simulink model "trainGate"  (R2014b)
settings: Solver=ode1  StartTime=0.0  StopTime=100  FixedStep=0.0001  MaxStep=0.0001  RelTol=1e-3
(part 1 of 2)
settings Model: Creator=sand080  LastModifiedBy=nall426
settings DataIOCC: LimitDataPoints=off
settings RTWCC: CustomInitializer=gettimeofday(&t0, 0);
settings RTWCC: CustomSourceCode=|
  | int gettimeofday(struct timeval * tp, struct timezone * tzp)
  | {
  |     // Note: some broken versions only have 8 trailing zero's, the correct epoch has 9 trailing zero's
  |     static const uint64_t EPOCH = ((uint64_t) 116444736000000000ULL);
  | 
  |     SYSTEMTIME  system_time;
  |     FILETIME    file_time;
  |     uint64_t    time;
  | 
  | 	GetSystemTime( &system_time );
  |     SystemTimeToFileTime( &system_time, &file_time );
  |     time =  ((uint64_t)file_time.dwLowDateTime )      ;
  |     time += ((uint64_t)file_time.dwHighDateTime) << 32;
  | 
  |     tp->tv_sec  = (long) ((time - EPOCH) / 10000000L);
  |     tp->tv_usec = (long) (system_time.wMilliseconds * 1000);
  |     return 0;
  | }
  | 
  | struct timeval t0, t1;
settings RTWCC: CustomHeaderCode=|
  | #include <stdint.h> // portable: uint64_t   MSVC: __int64
  | #include <Windows.h>
settings RTWCC: CustomTerminator=|
  | gettimeofday(&t1, 0);
  | 
  | long elapsed = (t1.tv_sec-t0.tv_sec)*1000000 + t1.tv_usec-t0.tv_usec;
  | printf("Time taken: %ld microseconds (%.3f seconds)\n", elapsed, (elapsed / 1000000.0));

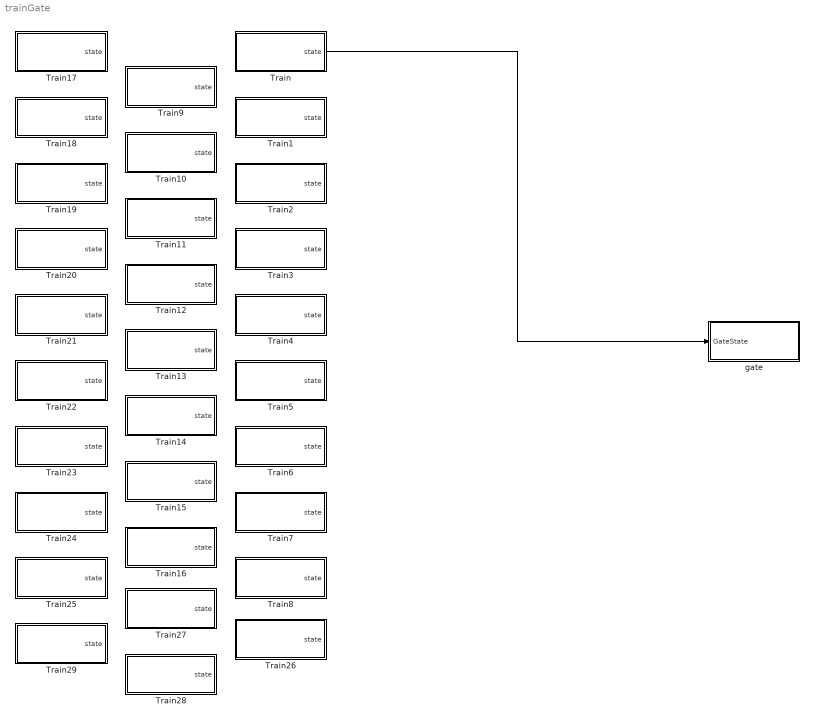
== system trainGate ==
  Train : Subsystem
  Train1 : Subsystem
  Train10 : Subsystem
  Train11 : Subsystem
  Train12 : Subsystem
  Train13 : Subsystem
  Train14 : Subsystem
  Train15 : Subsystem
  Train16 : Subsystem
  Train17 : Subsystem
  Train18 : Subsystem
  Train19 : Subsystem
  Train2 : Subsystem
  Train20 : Subsystem
  Train21 : Subsystem
  Train22 : Subsystem
  Train23 : Subsystem
  Train24 : Subsystem
  Train25 : Subsystem
  Train26 : Subsystem
  Train27 : Subsystem
  Train28 : Subsystem
  Train29 : Subsystem
  Train3 : Subsystem
  Train4 : Subsystem
  Train5 : Subsystem
  Train6 : Subsystem
  Train7 : Subsystem
  Train8 : Subsystem
  Train9 : Subsystem
  gate : Subsystem
  wires:
  Train/1(state) -> gate/1(GateState)

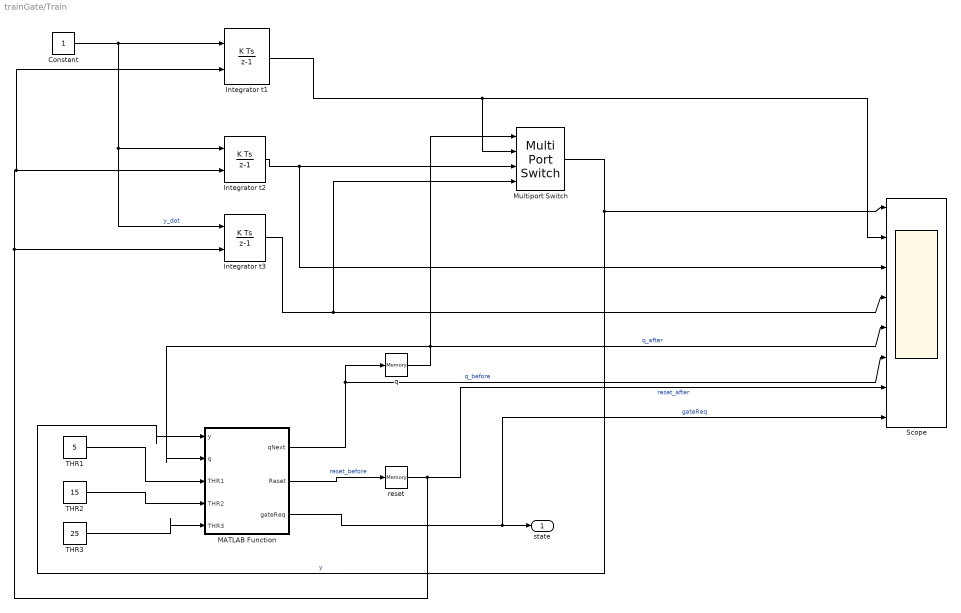
== system trainGate/Train ==
  Constant : Constant
  Integrator t1 : DiscreteIntegrator  ExternalReset=either  InitialConditionSetting=State (most efficient)  SampleTime=-1
  Integrator t2 : DiscreteIntegrator  ExternalReset=either  InitialCondition=5  InitialConditionSetting=State (most efficient)  SampleTime=-1
  Integrator t3 : DiscreteIntegrator  ExternalReset=either  InitialCondition=15  InitialConditionSetting=State (most efficient)  SampleTime=-1
  MATLAB Function : MATLAB Function  Priority=1  TreatAsAtomicUnit=on
  Multiport Switch : MultiPortSwitch
  Scope : Scope  NumInputPorts=8
      settings: TickLabels=on  ShowLegends=on  YMin=0~0~0~10~1~1~0~-1  YMax=40~20~20~30~3~3~1~1
  THR1 : Constant  Value=5
  THR2 : Constant  Value=15
  THR3 : Constant  Value=25
  q : Memory  X0=1  LinearizeMemory=on
  reset : Memory  X0=1  LinearizeMemory=on
  state : Outport
  wires:
  MATLAB Function/1(qNext) -> q/1, Scope/6  "q_before"
  Constant/1 -> Integrator t2/1, Integrator t3/1, Integrator t1/1  "y_dot"
  Integrator t2/1 -> Multiport Switch/3, Scope/3
  Integrator t1/1 -> Scope/2, Multiport Switch/2
  THR1/1 -> MATLAB Function/3(THR1)
  THR2/1 -> MATLAB Function/4(THR2)
  q/1 -> Multiport Switch/1, MATLAB Function/2(q), Scope/5  "q_after"
  THR3/1 -> MATLAB Function/5(THR3)
  Integrator t3/1 -> Multiport Switch/4, Scope/4
  MATLAB Function/2(Reset) -> reset/1  "reset_before"
  Multiport Switch/1 -> Scope/1, MATLAB Function/1(y)  "y"
  reset/1 -> Integrator t1/2, Integrator t2/2, Integrator t3/2, Scope/7  "reset_after"
  MATLAB Function/3(gateReq) -> Scope/8, state/1  "gateReq"

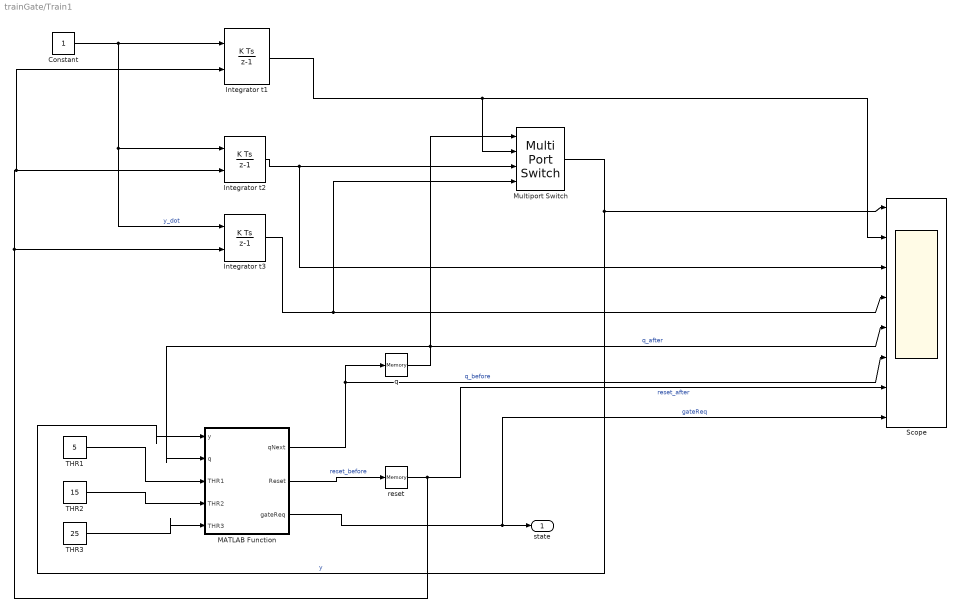
== system trainGate/Train1 ==
  Constant : Constant
  Integrator t1 : DiscreteIntegrator  ExternalReset=either  InitialConditionSetting=State (most efficient)  SampleTime=-1
  Integrator t2 : DiscreteIntegrator  ExternalReset=either  InitialCondition=5  InitialConditionSetting=State (most efficient)  SampleTime=-1
  Integrator t3 : DiscreteIntegrator  ExternalReset=either  InitialCondition=15  InitialConditionSetting=State (most efficient)  SampleTime=-1
  MATLAB Function : MATLAB Function  Priority=1  TreatAsAtomicUnit=on
  Multiport Switch : MultiPortSwitch
  Scope : Scope  NumInputPorts=8
      settings: TickLabels=on  ShowLegends=on  YMin=0~0~0~10~1~1~0~-1  YMax=40~20~20~30~3~3~1~1
  THR1 : Constant  Value=5
  THR2 : Constant  Value=15
  THR3 : Constant  Value=25
  q : Memory  X0=1  LinearizeMemory=on
  reset : Memory  X0=1  LinearizeMemory=on
  state : Outport
  wires:
  MATLAB Function/1(qNext) -> q/1, Scope/6  "q_before"
  Constant/1 -> Integrator t2/1, Integrator t3/1, Integrator t1/1  "y_dot"
  Integrator t2/1 -> Multiport Switch/3, Scope/3
  Integrator t1/1 -> Scope/2, Multiport Switch/2
  THR1/1 -> MATLAB Function/3(THR1)
  THR2/1 -> MATLAB Function/4(THR2)
  q/1 -> Multiport Switch/1, MATLAB Function/2(q), Scope/5  "q_after"
  THR3/1 -> MATLAB Function/5(THR3)
  Integrator t3/1 -> Multiport Switch/4, Scope/4
  MATLAB Function/2(Reset) -> reset/1  "reset_before"
  Multiport Switch/1 -> Scope/1, MATLAB Function/1(y)  "y"
  reset/1 -> Integrator t1/2, Integrator t2/2, Integrator t3/2, Scope/7  "reset_after"
  MATLAB Function/3(gateReq) -> Scope/8, state/1  "gateReq"

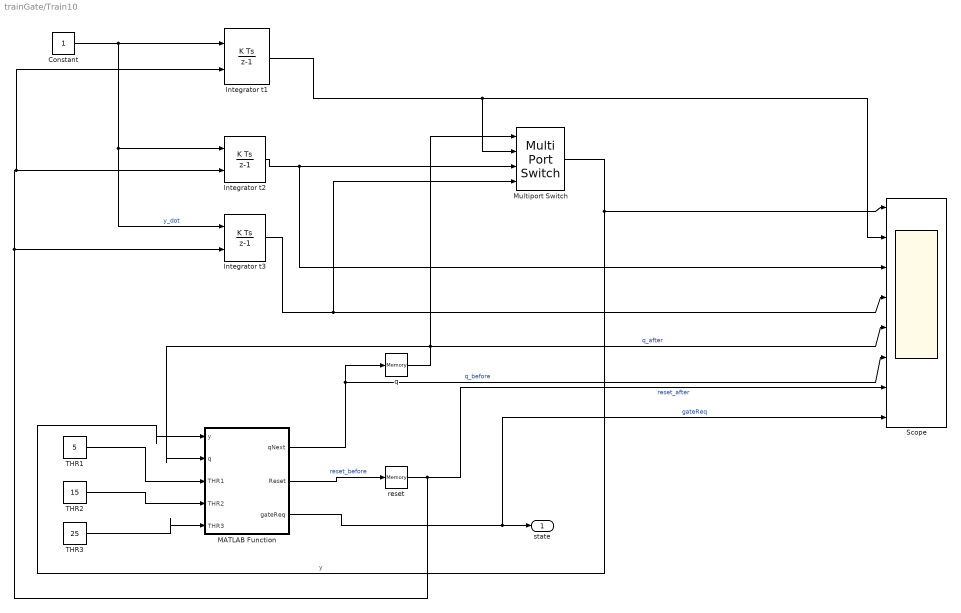
== system trainGate/Train10 ==
  Constant : Constant
  Integrator t1 : DiscreteIntegrator  ExternalReset=either  InitialConditionSetting=State (most efficient)  SampleTime=-1
  Integrator t2 : DiscreteIntegrator  ExternalReset=either  InitialCondition=5  InitialConditionSetting=State (most efficient)  SampleTime=-1
  Integrator t3 : DiscreteIntegrator  ExternalReset=either  InitialCondition=15  InitialConditionSetting=State (most efficient)  SampleTime=-1
  MATLAB Function : MATLAB Function  Priority=1  TreatAsAtomicUnit=on
  Multiport Switch : MultiPortSwitch
  Scope : Scope  NumInputPorts=8
      settings: TickLabels=on  ShowLegends=on  YMin=0~0~0~10~1~1~0~-1  YMax=40~20~20~30~3~3~1~1
  THR1 : Constant  Value=5
  THR2 : Constant  Value=15
  THR3 : Constant  Value=25
  q : Memory  X0=1  LinearizeMemory=on
  reset : Memory  X0=1  LinearizeMemory=on
  state : Outport
  wires:
  MATLAB Function/1(qNext) -> q/1, Scope/6  "q_before"
  Constant/1 -> Integrator t2/1, Integrator t3/1, Integrator t1/1  "y_dot"
  Integrator t2/1 -> Multiport Switch/3, Scope/3
  Integrator t1/1 -> Scope/2, Multiport Switch/2
  THR1/1 -> MATLAB Function/3(THR1)
  THR2/1 -> MATLAB Function/4(THR2)
  q/1 -> Multiport Switch/1, MATLAB Function/2(q), Scope/5  "q_after"
  THR3/1 -> MATLAB Function/5(THR3)
  Integrator t3/1 -> Multiport Switch/4, Scope/4
  MATLAB Function/2(Reset) -> reset/1  "reset_before"
  Multiport Switch/1 -> Scope/1, MATLAB Function/1(y)  "y"
  reset/1 -> Integrator t1/2, Integrator t2/2, Integrator t3/2, Scope/7  "reset_after"
  MATLAB Function/3(gateReq) -> Scope/8, state/1  "gateReq"

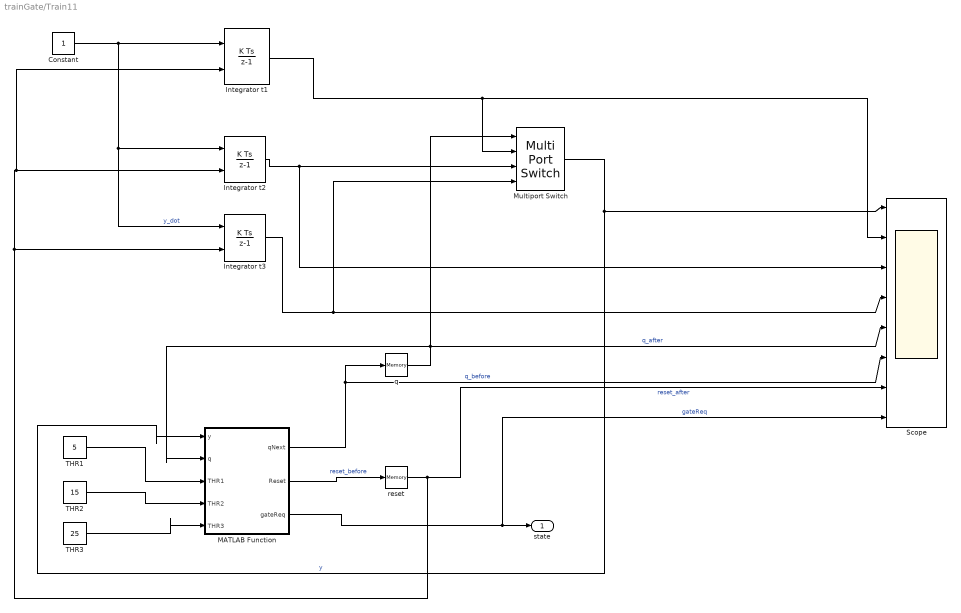
== system trainGate/Train11 ==
  Constant : Constant
  Integrator t1 : DiscreteIntegrator  ExternalReset=either  InitialConditionSetting=State (most efficient)  SampleTime=-1
  Integrator t2 : DiscreteIntegrator  ExternalReset=either  InitialCondition=5  InitialConditionSetting=State (most efficient)  SampleTime=-1
  Integrator t3 : DiscreteIntegrator  ExternalReset=either  InitialCondition=15  InitialConditionSetting=State (most efficient)  SampleTime=-1
  MATLAB Function : MATLAB Function  Priority=1  TreatAsAtomicUnit=on
  Multiport Switch : MultiPortSwitch
  Scope : Scope  NumInputPorts=8
      settings: TickLabels=on  ShowLegends=on  YMin=0~0~0~10~1~1~0~-1  YMax=40~20~20~30~3~3~1~1
  THR1 : Constant  Value=5
  THR2 : Constant  Value=15
  THR3 : Constant  Value=25
  q : Memory  X0=1  LinearizeMemory=on
  reset : Memory  X0=1  LinearizeMemory=on
  state : Outport
  wires:
  MATLAB Function/1(qNext) -> q/1, Scope/6  "q_before"
  Constant/1 -> Integrator t2/1, Integrator t3/1, Integrator t1/1  "y_dot"
  Integrator t2/1 -> Multiport Switch/3, Scope/3
  Integrator t1/1 -> Scope/2, Multiport Switch/2
  THR1/1 -> MATLAB Function/3(THR1)
  THR2/1 -> MATLAB Function/4(THR2)
  q/1 -> Multiport Switch/1, MATLAB Function/2(q), Scope/5  "q_after"
  THR3/1 -> MATLAB Function/5(THR3)
  Integrator t3/1 -> Multiport Switch/4, Scope/4
  MATLAB Function/2(Reset) -> reset/1  "reset_before"
  Multiport Switch/1 -> Scope/1, MATLAB Function/1(y)  "y"
  reset/1 -> Integrator t1/2, Integrator t2/2, Integrator t3/2, Scope/7  "reset_after"
  MATLAB Function/3(gateReq) -> Scope/8, state/1  "gateReq"

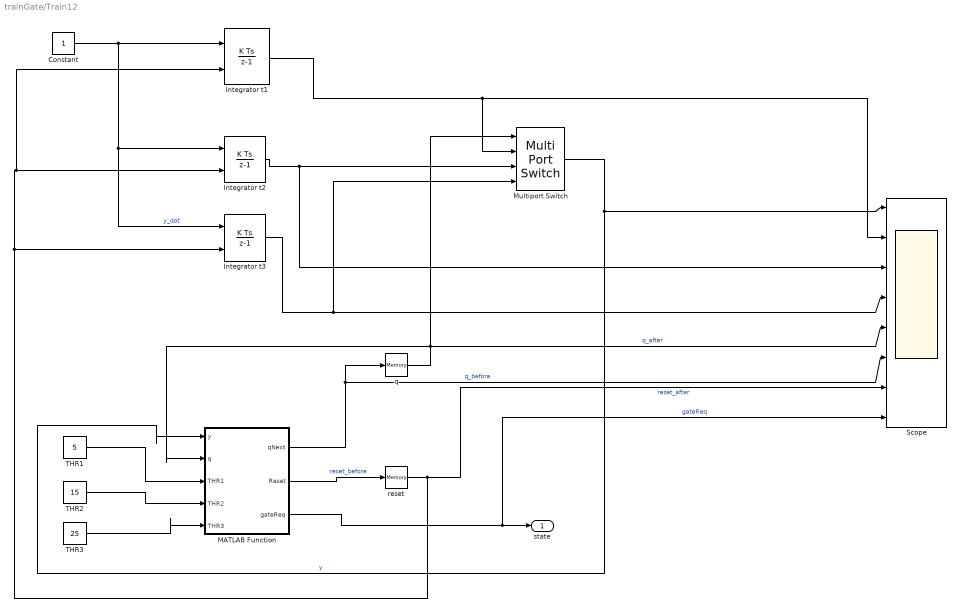
== system trainGate/Train12 ==
  Constant : Constant
  Integrator t1 : DiscreteIntegrator  ExternalReset=either  InitialConditionSetting=State (most efficient)  SampleTime=-1
  Integrator t2 : DiscreteIntegrator  ExternalReset=either  InitialCondition=5  InitialConditionSetting=State (most efficient)  SampleTime=-1
  Integrator t3 : DiscreteIntegrator  ExternalReset=either  InitialCondition=15  InitialConditionSetting=State (most efficient)  SampleTime=-1
  MATLAB Function : MATLAB Function  Priority=1  TreatAsAtomicUnit=on
  Multiport Switch : MultiPortSwitch
  Scope : Scope  NumInputPorts=8
      settings: TickLabels=on  ShowLegends=on  YMin=0~0~0~10~1~1~0~-1  YMax=40~20~20~30~3~3~1~1
  THR1 : Constant  Value=5
  THR2 : Constant  Value=15
  THR3 : Constant  Value=25
  q : Memory  X0=1  LinearizeMemory=on
  reset : Memory  X0=1  LinearizeMemory=on
  state : Outport
  wires:
  MATLAB Function/1(qNext) -> q/1, Scope/6  "q_before"
  Constant/1 -> Integrator t2/1, Integrator t3/1, Integrator t1/1  "y_dot"
  Integrator t2/1 -> Multiport Switch/3, Scope/3
  Integrator t1/1 -> Scope/2, Multiport Switch/2
  THR1/1 -> MATLAB Function/3(THR1)
  THR2/1 -> MATLAB Function/4(THR2)
  q/1 -> Multiport Switch/1, MATLAB Function/2(q), Scope/5  "q_after"
  THR3/1 -> MATLAB Function/5(THR3)
  Integrator t3/1 -> Multiport Switch/4, Scope/4
  MATLAB Function/2(Reset) -> reset/1  "reset_before"
  Multiport Switch/1 -> Scope/1, MATLAB Function/1(y)  "y"
  reset/1 -> Integrator t1/2, Integrator t2/2, Integrator t3/2, Scope/7  "reset_after"
  MATLAB Function/3(gateReq) -> Scope/8, state/1  "gateReq"

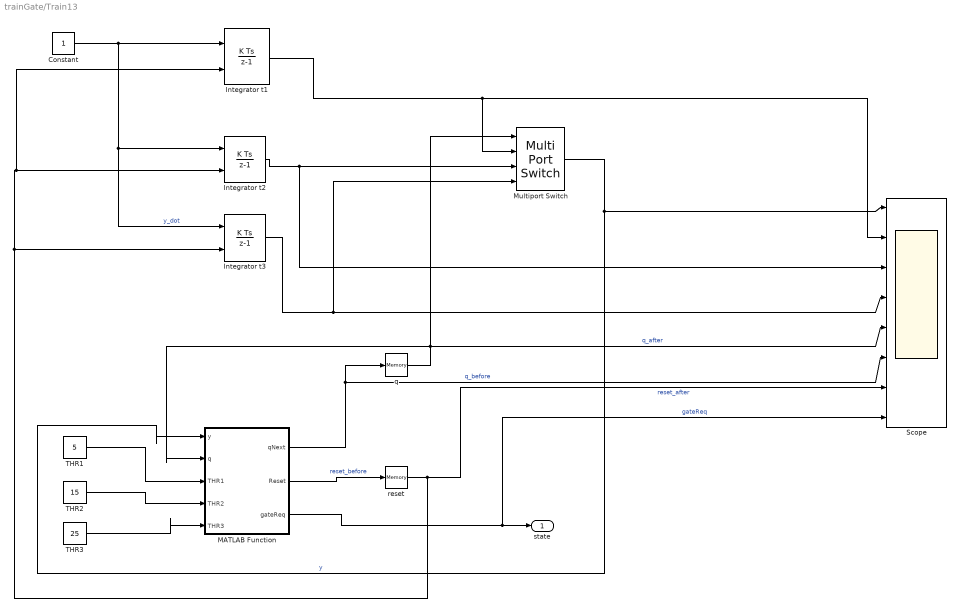
== system trainGate/Train13 ==
  Constant : Constant
  Integrator t1 : DiscreteIntegrator  ExternalReset=either  InitialConditionSetting=State (most efficient)  SampleTime=-1
  Integrator t2 : DiscreteIntegrator  ExternalReset=either  InitialCondition=5  InitialConditionSetting=State (most efficient)  SampleTime=-1
  Integrator t3 : DiscreteIntegrator  ExternalReset=either  InitialCondition=15  InitialConditionSetting=State (most efficient)  SampleTime=-1
  MATLAB Function : MATLAB Function  Priority=1  TreatAsAtomicUnit=on
  Multiport Switch : MultiPortSwitch
  Scope : Scope  NumInputPorts=8
      settings: TickLabels=on  ShowLegends=on  YMin=0~0~0~10~1~1~0~-1  YMax=40~20~20~30~3~3~1~1
  THR1 : Constant  Value=5
  THR2 : Constant  Value=15
  THR3 : Constant  Value=25
  q : Memory  X0=1  LinearizeMemory=on
  reset : Memory  X0=1  LinearizeMemory=on
  state : Outport
  wires:
  MATLAB Function/1(qNext) -> q/1, Scope/6  "q_before"
  Constant/1 -> Integrator t2/1, Integrator t3/1, Integrator t1/1  "y_dot"
  Integrator t2/1 -> Multiport Switch/3, Scope/3
  Integrator t1/1 -> Scope/2, Multiport Switch/2
  THR1/1 -> MATLAB Function/3(THR1)
  THR2/1 -> MATLAB Function/4(THR2)
  q/1 -> Multiport Switch/1, MATLAB Function/2(q), Scope/5  "q_after"
  THR3/1 -> MATLAB Function/5(THR3)
  Integrator t3/1 -> Multiport Switch/4, Scope/4
  MATLAB Function/2(Reset) -> reset/1  "reset_before"
  Multiport Switch/1 -> Scope/1, MATLAB Function/1(y)  "y"
  reset/1 -> Integrator t1/2, Integrator t2/2, Integrator t3/2, Scope/7  "reset_after"
  MATLAB Function/3(gateReq) -> Scope/8, state/1  "gateReq"

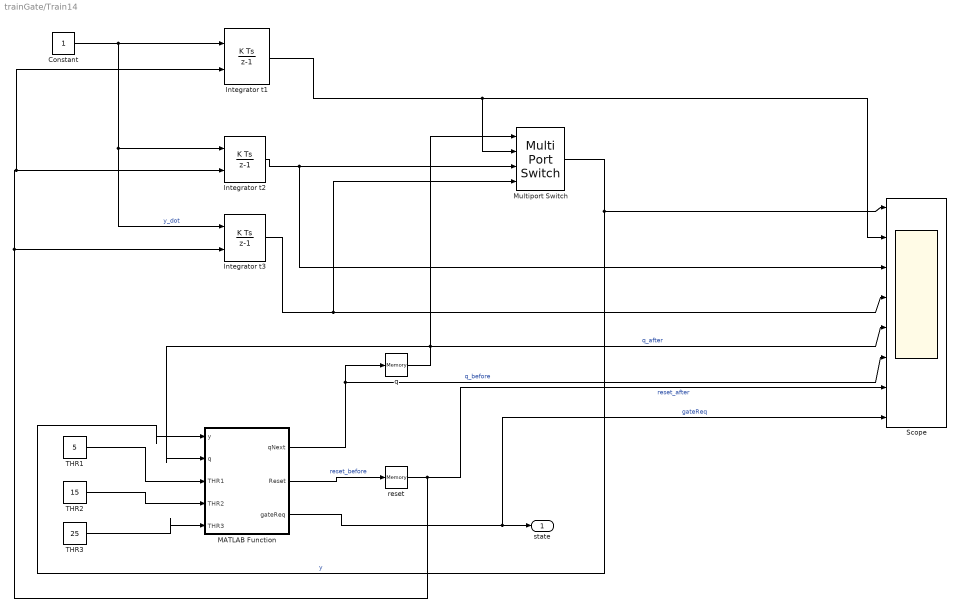
== system trainGate/Train14 ==
  Constant : Constant
  Integrator t1 : DiscreteIntegrator  ExternalReset=either  InitialConditionSetting=State (most efficient)  SampleTime=-1
  Integrator t2 : DiscreteIntegrator  ExternalReset=either  InitialCondition=5  InitialConditionSetting=State (most efficient)  SampleTime=-1
  Integrator t3 : DiscreteIntegrator  ExternalReset=either  InitialCondition=15  InitialConditionSetting=State (most efficient)  SampleTime=-1
  MATLAB Function : MATLAB Function  Priority=1  TreatAsAtomicUnit=on
  Multiport Switch : MultiPortSwitch
  Scope : Scope  NumInputPorts=8
      settings: TickLabels=on  ShowLegends=on  YMin=0~0~0~10~1~1~0~-1  YMax=40~20~20~30~3~3~1~1
  THR1 : Constant  Value=5
  THR2 : Constant  Value=15
  THR3 : Constant  Value=25
  q : Memory  X0=1  LinearizeMemory=on
  reset : Memory  X0=1  LinearizeMemory=on
  state : Outport
  wires:
  MATLAB Function/1(qNext) -> q/1, Scope/6  "q_before"
  Constant/1 -> Integrator t2/1, Integrator t3/1, Integrator t1/1  "y_dot"
  Integrator t2/1 -> Multiport Switch/3, Scope/3
  Integrator t1/1 -> Scope/2, Multiport Switch/2
  THR1/1 -> MATLAB Function/3(THR1)
  THR2/1 -> MATLAB Function/4(THR2)
  q/1 -> Multiport Switch/1, MATLAB Function/2(q), Scope/5  "q_after"
  THR3/1 -> MATLAB Function/5(THR3)
  Integrator t3/1 -> Multiport Switch/4, Scope/4
  MATLAB Function/2(Reset) -> reset/1  "reset_before"
  Multiport Switch/1 -> Scope/1, MATLAB Function/1(y)  "y"
  reset/1 -> Integrator t1/2, Integrator t2/2, Integrator t3/2, Scope/7  "reset_after"
  MATLAB Function/3(gateReq) -> Scope/8, state/1  "gateReq"

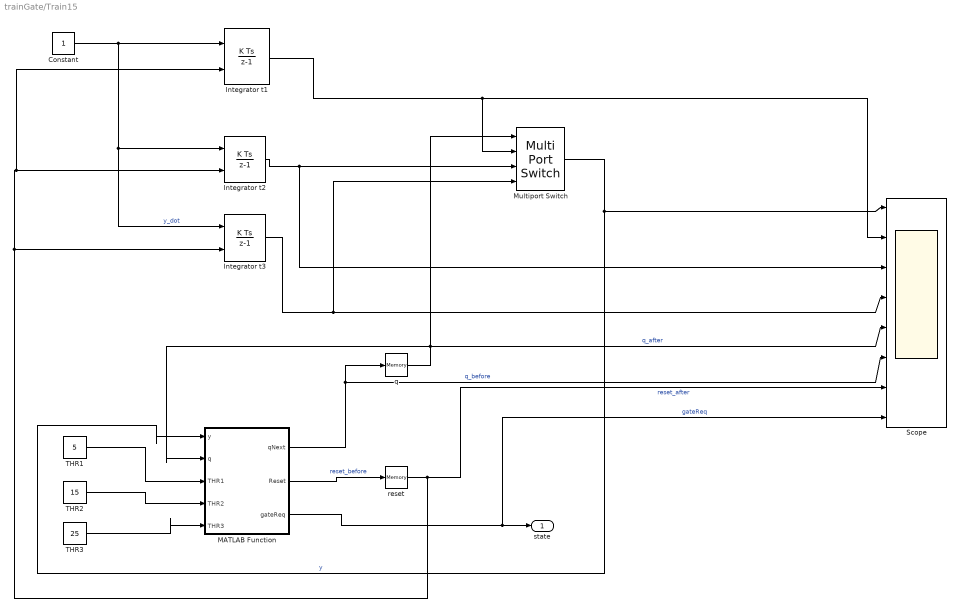
== system trainGate/Train15 ==
  Constant : Constant
  Integrator t1 : DiscreteIntegrator  ExternalReset=either  InitialConditionSetting=State (most efficient)  SampleTime=-1
  Integrator t2 : DiscreteIntegrator  ExternalReset=either  InitialCondition=5  InitialConditionSetting=State (most efficient)  SampleTime=-1
  Integrator t3 : DiscreteIntegrator  ExternalReset=either  InitialCondition=15  InitialConditionSetting=State (most efficient)  SampleTime=-1
  MATLAB Function : MATLAB Function  Priority=1  TreatAsAtomicUnit=on
  Multiport Switch : MultiPortSwitch
  Scope : Scope  NumInputPorts=8
      settings: TickLabels=on  ShowLegends=on  YMin=0~0~0~10~1~1~0~-1  YMax=40~20~20~30~3~3~1~1
  THR1 : Constant  Value=5
  THR2 : Constant  Value=15
  THR3 : Constant  Value=25
  q : Memory  X0=1  LinearizeMemory=on
  reset : Memory  X0=1  LinearizeMemory=on
  state : Outport
  wires:
  MATLAB Function/1(qNext) -> q/1, Scope/6  "q_before"
  Constant/1 -> Integrator t2/1, Integrator t3/1, Integrator t1/1  "y_dot"
  Integrator t2/1 -> Multiport Switch/3, Scope/3
  Integrator t1/1 -> Scope/2, Multiport Switch/2
  THR1/1 -> MATLAB Function/3(THR1)
  THR2/1 -> MATLAB Function/4(THR2)
  q/1 -> Multiport Switch/1, MATLAB Function/2(q), Scope/5  "q_after"
  THR3/1 -> MATLAB Function/5(THR3)
  Integrator t3/1 -> Multiport Switch/4, Scope/4
  MATLAB Function/2(Reset) -> reset/1  "reset_before"
  Multiport Switch/1 -> Scope/1, MATLAB Function/1(y)  "y"
  reset/1 -> Integrator t1/2, Integrator t2/2, Integrator t3/2, Scope/7  "reset_after"
  MATLAB Function/3(gateReq) -> Scope/8, state/1  "gateReq"

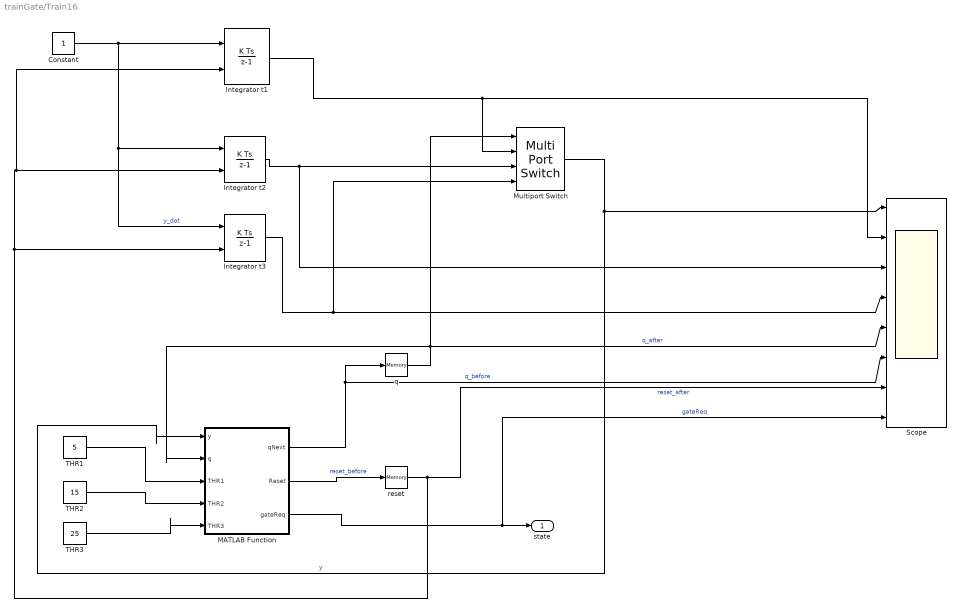
== system trainGate/Train16 ==
  Constant : Constant
  Integrator t1 : DiscreteIntegrator  ExternalReset=either  InitialConditionSetting=State (most efficient)  SampleTime=-1
  Integrator t2 : DiscreteIntegrator  ExternalReset=either  InitialCondition=5  InitialConditionSetting=State (most efficient)  SampleTime=-1
  Integrator t3 : DiscreteIntegrator  ExternalReset=either  InitialCondition=15  InitialConditionSetting=State (most efficient)  SampleTime=-1
  MATLAB Function : MATLAB Function  Priority=1  TreatAsAtomicUnit=on
  Multiport Switch : MultiPortSwitch
  Scope : Scope  NumInputPorts=8
      settings: TickLabels=on  ShowLegends=on  YMin=0~0~0~10~1~1~0~-1  YMax=40~20~20~30~3~3~1~1
  THR1 : Constant  Value=5
  THR2 : Constant  Value=15
  THR3 : Constant  Value=25
  q : Memory  X0=1  LinearizeMemory=on
  reset : Memory  X0=1  LinearizeMemory=on
  state : Outport
  wires:
  MATLAB Function/1(qNext) -> q/1, Scope/6  "q_before"
  Constant/1 -> Integrator t2/1, Integrator t3/1, Integrator t1/1  "y_dot"
  Integrator t2/1 -> Multiport Switch/3, Scope/3
  Integrator t1/1 -> Scope/2, Multiport Switch/2
  THR1/1 -> MATLAB Function/3(THR1)
  THR2/1 -> MATLAB Function/4(THR2)
  q/1 -> Multiport Switch/1, MATLAB Function/2(q), Scope/5  "q_after"
  THR3/1 -> MATLAB Function/5(THR3)
  Integrator t3/1 -> Multiport Switch/4, Scope/4
  MATLAB Function/2(Reset) -> reset/1  "reset_before"
  Multiport Switch/1 -> Scope/1, MATLAB Function/1(y)  "y"
  reset/1 -> Integrator t1/2, Integrator t2/2, Integrator t3/2, Scope/7  "reset_after"
  MATLAB Function/3(gateReq) -> Scope/8, state/1  "gateReq"

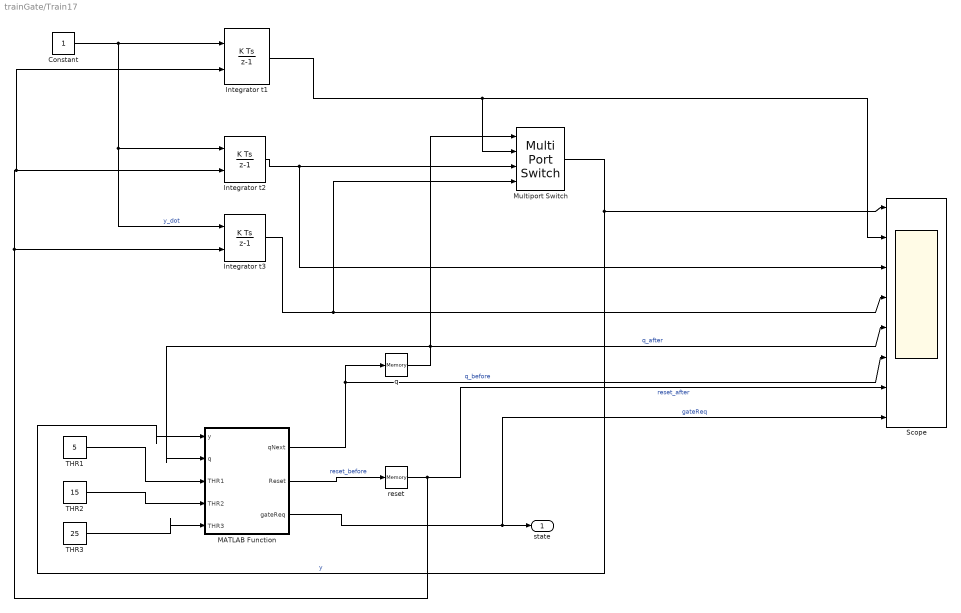
== system trainGate/Train17 ==
  Constant : Constant
  Integrator t1 : DiscreteIntegrator  ExternalReset=either  InitialConditionSetting=State (most efficient)  SampleTime=-1
  Integrator t2 : DiscreteIntegrator  ExternalReset=either  InitialCondition=5  InitialConditionSetting=State (most efficient)  SampleTime=-1
  Integrator t3 : DiscreteIntegrator  ExternalReset=either  InitialCondition=15  InitialConditionSetting=State (most efficient)  SampleTime=-1
  MATLAB Function : MATLAB Function  Priority=1  TreatAsAtomicUnit=on
  Multiport Switch : MultiPortSwitch
  Scope : Scope  NumInputPorts=8
      settings: TickLabels=on  ShowLegends=on  YMin=0~0~0~10~1~1~0~-1  YMax=40~20~20~30~3~3~1~1
  THR1 : Constant  Value=5
  THR2 : Constant  Value=15
  THR3 : Constant  Value=25
  q : Memory  X0=1  LinearizeMemory=on
  reset : Memory  X0=1  LinearizeMemory=on
  state : Outport
  wires:
  MATLAB Function/1(qNext) -> q/1, Scope/6  "q_before"
  Constant/1 -> Integrator t2/1, Integrator t3/1, Integrator t1/1  "y_dot"
  Integrator t2/1 -> Multiport Switch/3, Scope/3
  Integrator t1/1 -> Scope/2, Multiport Switch/2
  THR1/1 -> MATLAB Function/3(THR1)
  THR2/1 -> MATLAB Function/4(THR2)
  q/1 -> Multiport Switch/1, MATLAB Function/2(q), Scope/5  "q_after"
  THR3/1 -> MATLAB Function/5(THR3)
  Integrator t3/1 -> Multiport Switch/4, Scope/4
  MATLAB Function/2(Reset) -> reset/1  "reset_before"
  Multiport Switch/1 -> Scope/1, MATLAB Function/1(y)  "y"
  reset/1 -> Integrator t1/2, Integrator t2/2, Integrator t3/2, Scope/7  "reset_after"
  MATLAB Function/3(gateReq) -> Scope/8, state/1  "gateReq"

== system trainGate/Train18 ==
  Constant : Constant
  Integrator t1 : DiscreteIntegrator  ExternalReset=either  InitialConditionSetting=State (most efficient)  SampleTime=-1
  Integrator t2 : DiscreteIntegrator  ExternalReset=either  InitialCondition=5  InitialConditionSetting=State (most efficient)  SampleTime=-1
  Integrator t3 : DiscreteIntegrator  ExternalReset=either  InitialCondition=15  InitialConditionSetting=State (most efficient)  SampleTime=-1
  MATLAB Function : MATLAB Function  Priority=1  TreatAsAtomicUnit=on
  Multiport Switch : MultiPortSwitch
  Scope : Scope  NumInputPorts=8
      settings: TickLabels=on  ShowLegends=on  YMin=0~0~0~10~1~1~0~-1  YMax=40~20~20~30~3~3~1~1
  THR1 : Constant  Value=5
  THR2 : Constant  Value=15
  THR3 : Constant  Value=25
  q : Memory  X0=1  LinearizeMemory=on
  reset : Memory  X0=1  LinearizeMemory=on
  state : Outport
  wires:
  MATLAB Function/1(qNext) -> q/1, Scope/6  "q_before"
  Constant/1 -> Integrator t2/1, Integrator t3/1, Integrator t1/1  "y_dot"
  Integrator t2/1 -> Multiport Switch/3, Scope/3
  Integrator t1/1 -> Scope/2, Multiport Switch/2
  THR1/1 -> MATLAB Function/3(THR1)
  THR2/1 -> MATLAB Function/4(THR2)
  q/1 -> Multiport Switch/1, MATLAB Function/2(q), Scope/5  "q_after"
  THR3/1 -> MATLAB Function/5(THR3)
  Integrator t3/1 -> Multiport Switch/4, Scope/4
  MATLAB Function/2(Reset) -> reset/1  "reset_before"
  Multiport Switch/1 -> Scope/1, MATLAB Function/1(y)  "y"
  reset/1 -> Integrator t1/2, Integrator t2/2, Integrator t3/2, Scope/7  "reset_after"
  MATLAB Function/3(gateReq) -> Scope/8, state/1  "gateReq"

== system trainGate/Train19 ==
  Constant : Constant
  Integrator t1 : DiscreteIntegrator  ExternalReset=either  InitialConditionSetting=State (most efficient)  SampleTime=-1
  Integrator t2 : DiscreteIntegrator  ExternalReset=either  InitialCondition=5  InitialConditionSetting=State (most efficient)  SampleTime=-1
  Integrator t3 : DiscreteIntegrator  ExternalReset=either  InitialCondition=15  InitialConditionSetting=State (most efficient)  SampleTime=-1
  MATLAB Function : MATLAB Function  Priority=1  TreatAsAtomicUnit=on
  Multiport Switch : MultiPortSwitch
  Scope : Scope  NumInputPorts=8
      settings: TickLabels=on  ShowLegends=on  YMin=0~0~0~10~1~1~0~-1  YMax=40~20~20~30~3~3~1~1
  THR1 : Constant  Value=5
  THR2 : Constant  Value=15
  THR3 : Constant  Value=25
  q : Memory  X0=1  LinearizeMemory=on
  reset : Memory  X0=1  LinearizeMemory=on
  state : Outport
  wires:
  MATLAB Function/1(qNext) -> q/1, Scope/6  "q_before"
  Constant/1 -> Integrator t2/1, Integrator t3/1, Integrator t1/1  "y_dot"
  Integrator t2/1 -> Multiport Switch/3, Scope/3
  Integrator t1/1 -> Scope/2, Multiport Switch/2
  THR1/1 -> MATLAB Function/3(THR1)
  THR2/1 -> MATLAB Function/4(THR2)
  q/1 -> Multiport Switch/1, MATLAB Function/2(q), Scope/5  "q_after"
  THR3/1 -> MATLAB Function/5(THR3)
  Integrator t3/1 -> Multiport Switch/4, Scope/4
  MATLAB Function/2(Reset) -> reset/1  "reset_before"
  Multiport Switch/1 -> Scope/1, MATLAB Function/1(y)  "y"
  reset/1 -> Integrator t1/2, Integrator t2/2, Integrator t3/2, Scope/7  "reset_after"
  MATLAB Function/3(gateReq) -> Scope/8, state/1  "gateReq"

== system trainGate/Train2 ==
  Constant : Constant
  Integrator t1 : DiscreteIntegrator  ExternalReset=either  InitialConditionSetting=State (most efficient)  SampleTime=-1
  Integrator t2 : DiscreteIntegrator  ExternalReset=either  InitialCondition=5  InitialConditionSetting=State (most efficient)  SampleTime=-1
  Integrator t3 : DiscreteIntegrator  ExternalReset=either  InitialCondition=15  InitialConditionSetting=State (most efficient)  SampleTime=-1
  MATLAB Function : MATLAB Function  Priority=1  TreatAsAtomicUnit=on
  Multiport Switch : MultiPortSwitch
  Scope : Scope  NumInputPorts=8
      settings: TickLabels=on  ShowLegends=on  YMin=0~0~0~10~1~1~0~-1  YMax=40~20~20~30~3~3~1~1
  THR1 : Constant  Value=5
  THR2 : Constant  Value=15
  THR3 : Constant  Value=25
  q : Memory  X0=1  LinearizeMemory=on
  reset : Memory  X0=1  LinearizeMemory=on
  state : Outport
  wires:
  MATLAB Function/1(qNext) -> q/1, Scope/6  "q_before"
  Constant/1 -> Integrator t2/1, Integrator t3/1, Integrator t1/1  "y_dot"
  Integrator t2/1 -> Multiport Switch/3, Scope/3
  Integrator t1/1 -> Scope/2, Multiport Switch/2
  THR1/1 -> MATLAB Function/3(THR1)
  THR2/1 -> MATLAB Function/4(THR2)
  q/1 -> Multiport Switch/1, MATLAB Function/2(q), Scope/5  "q_after"
  THR3/1 -> MATLAB Function/5(THR3)
  Integrator t3/1 -> Multiport Switch/4, Scope/4
  MATLAB Function/2(Reset) -> reset/1  "reset_before"
  Multiport Switch/1 -> Scope/1, MATLAB Function/1(y)  "y"
  reset/1 -> Integrator t1/2, Integrator t2/2, Integrator t3/2, Scope/7  "reset_after"
  MATLAB Function/3(gateReq) -> Scope/8, state/1  "gateReq"

== system trainGate/Train20 ==
  Constant : Constant
  Integrator t1 : DiscreteIntegrator  ExternalReset=either  InitialConditionSetting=State (most efficient)  SampleTime=-1
  Integrator t2 : DiscreteIntegrator  ExternalReset=either  InitialCondition=5  InitialConditionSetting=State (most efficient)  SampleTime=-1
  Integrator t3 : DiscreteIntegrator  ExternalReset=either  InitialCondition=15  InitialConditionSetting=State (most efficient)  SampleTime=-1
  MATLAB Function : MATLAB Function  Priority=1  TreatAsAtomicUnit=on
  Multiport Switch : MultiPortSwitch
  Scope : Scope  NumInputPorts=8
      settings: TickLabels=on  ShowLegends=on  YMin=0~0~0~10~1~1~0~-1  YMax=40~20~20~30~3~3~1~1
  THR1 : Constant  Value=5
  THR2 : Constant  Value=15
  THR3 : Constant  Value=25
  q : Memory  X0=1  LinearizeMemory=on
  reset : Memory  X0=1  LinearizeMemory=on
  state : Outport
  wires:
  MATLAB Function/1(qNext) -> q/1, Scope/6  "q_before"
  Constant/1 -> Integrator t2/1, Integrator t3/1, Integrator t1/1  "y_dot"
  Integrator t2/1 -> Multiport Switch/3, Scope/3
  Integrator t1/1 -> Scope/2, Multiport Switch/2
  THR1/1 -> MATLAB Function/3(THR1)
  THR2/1 -> MATLAB Function/4(THR2)
  q/1 -> Multiport Switch/1, MATLAB Function/2(q), Scope/5  "q_after"
  THR3/1 -> MATLAB Function/5(THR3)
  Integrator t3/1 -> Multiport Switch/4, Scope/4
  MATLAB Function/2(Reset) -> reset/1  "reset_before"
  Multiport Switch/1 -> Scope/1, MATLAB Function/1(y)  "y"
  reset/1 -> Integrator t1/2, Integrator t2/2, Integrator t3/2, Scope/7  "reset_after"
  MATLAB Function/3(gateReq) -> Scope/8, state/1  "gateReq"

== system trainGate/Train21 ==
  Constant : Constant
  Integrator t1 : DiscreteIntegrator  ExternalReset=either  InitialConditionSetting=State (most efficient)  SampleTime=-1
  Integrator t2 : DiscreteIntegrator  ExternalReset=either  InitialCondition=5  InitialConditionSetting=State (most efficient)  SampleTime=-1
  Integrator t3 : DiscreteIntegrator  ExternalReset=either  InitialCondition=15  InitialConditionSetting=State (most efficient)  SampleTime=-1
  MATLAB Function : MATLAB Function  Priority=1  TreatAsAtomicUnit=on
  Multiport Switch : MultiPortSwitch
  Scope : Scope  NumInputPorts=8
      settings: TickLabels=on  ShowLegends=on  YMin=0~0~0~10~1~1~0~-1  YMax=40~20~20~30~3~3~1~1
  THR1 : Constant  Value=5
  THR2 : Constant  Value=15
  THR3 : Constant  Value=25
  q : Memory  X0=1  LinearizeMemory=on
  reset : Memory  X0=1  LinearizeMemory=on
  state : Outport
  wires:
  MATLAB Function/1(qNext) -> q/1, Scope/6  "q_before"
  Constant/1 -> Integrator t2/1, Integrator t3/1, Integrator t1/1  "y_dot"
  Integrator t2/1 -> Multiport Switch/3, Scope/3
  Integrator t1/1 -> Scope/2, Multiport Switch/2
  THR1/1 -> MATLAB Function/3(THR1)
  THR2/1 -> MATLAB Function/4(THR2)
  q/1 -> Multiport Switch/1, MATLAB Function/2(q), Scope/5  "q_after"
  THR3/1 -> MATLAB Function/5(THR3)
  Integrator t3/1 -> Multiport Switch/4, Scope/4
  MATLAB Function/2(Reset) -> reset/1  "reset_before"
  Multiport Switch/1 -> Scope/1, MATLAB Function/1(y)  "y"
  reset/1 -> Integrator t1/2, Integrator t2/2, Integrator t3/2, Scope/7  "reset_after"
  MATLAB Function/3(gateReq) -> Scope/8, state/1  "gateReq"

== system trainGate/Train22 ==
  Constant : Constant
  Integrator t1 : DiscreteIntegrator  ExternalReset=either  InitialConditionSetting=State (most efficient)  SampleTime=-1
  Integrator t2 : DiscreteIntegrator  ExternalReset=either  InitialCondition=5  InitialConditionSetting=State (most efficient)  SampleTime=-1
  Integrator t3 : DiscreteIntegrator  ExternalReset=either  InitialCondition=15  InitialConditionSetting=State (most efficient)  SampleTime=-1
  MATLAB Function : MATLAB Function  Priority=1  TreatAsAtomicUnit=on
  Multiport Switch : MultiPortSwitch
  Scope : Scope  NumInputPorts=8
      settings: TickLabels=on  ShowLegends=on  YMin=0~0~0~10~1~1~0~-1  YMax=40~20~20~30~3~3~1~1
  THR1 : Constant  Value=5
  THR2 : Constant  Value=15
  THR3 : Constant  Value=25
  q : Memory  X0=1  LinearizeMemory=on
  reset : Memory  X0=1  LinearizeMemory=on
  state : Outport
  wires:
  MATLAB Function/1(qNext) -> q/1, Scope/6  "q_before"
  Constant/1 -> Integrator t2/1, Integrator t3/1, Integrator t1/1  "y_dot"
  Integrator t2/1 -> Multiport Switch/3, Scope/3
  Integrator t1/1 -> Scope/2, Multiport Switch/2
  THR1/1 -> MATLAB Function/3(THR1)
  THR2/1 -> MATLAB Function/4(THR2)
  q/1 -> Multiport Switch/1, MATLAB Function/2(q), Scope/5  "q_after"
  THR3/1 -> MATLAB Function/5(THR3)
  Integrator t3/1 -> Multiport Switch/4, Scope/4
  MATLAB Function/2(Reset) -> reset/1  "reset_before"
  Multiport Switch/1 -> Scope/1, MATLAB Function/1(y)  "y"
  reset/1 -> Integrator t1/2, Integrator t2/2, Integrator t3/2, Scope/7  "reset_after"
  MATLAB Function/3(gateReq) -> Scope/8, state/1  "gateReq"

== system trainGate/Train23 ==
  Constant : Constant
  Integrator t1 : DiscreteIntegrator  ExternalReset=either  InitialConditionSetting=State (most efficient)  SampleTime=-1
  Integrator t2 : DiscreteIntegrator  ExternalReset=either  InitialCondition=5  InitialConditionSetting=State (most efficient)  SampleTime=-1
  Integrator t3 : DiscreteIntegrator  ExternalReset=either  InitialCondition=15  InitialConditionSetting=State (most efficient)  SampleTime=-1
  MATLAB Function : MATLAB Function  Priority=1  TreatAsAtomicUnit=on
  Multiport Switch : MultiPortSwitch
  Scope : Scope  NumInputPorts=8
      settings: TickLabels=on  ShowLegends=on  YMin=0~0~0~10~1~1~0~-1  YMax=40~20~20~30~3~3~1~1
  THR1 : Constant  Value=5
  THR2 : Constant  Value=15
  THR3 : Constant  Value=25
  q : Memory  X0=1  LinearizeMemory=on
  reset : Memory  X0=1  LinearizeMemory=on
  state : Outport
  wires:
  MATLAB Function/1(qNext) -> q/1, Scope/6  "q_before"
  Constant/1 -> Integrator t2/1, Integrator t3/1, Integrator t1/1  "y_dot"
  Integrator t2/1 -> Multiport Switch/3, Scope/3
  Integrator t1/1 -> Scope/2, Multiport Switch/2
  THR1/1 -> MATLAB Function/3(THR1)
  THR2/1 -> MATLAB Function/4(THR2)
  q/1 -> Multiport Switch/1, MATLAB Function/2(q), Scope/5  "q_after"
  THR3/1 -> MATLAB Function/5(THR3)
  Integrator t3/1 -> Multiport Switch/4, Scope/4
  MATLAB Function/2(Reset) -> reset/1  "reset_before"
  Multiport Switch/1 -> Scope/1, MATLAB Function/1(y)  "y"
  reset/1 -> Integrator t1/2, Integrator t2/2, Integrator t3/2, Scope/7  "reset_after"
  MATLAB Function/3(gateReq) -> Scope/8, state/1  "gateReq"

== system trainGate/Train24 ==
  Constant : Constant
  Integrator t1 : DiscreteIntegrator  ExternalReset=either  InitialConditionSetting=State (most efficient)  SampleTime=-1
  Integrator t2 : DiscreteIntegrator  ExternalReset=either  InitialCondition=5  InitialConditionSetting=State (most efficient)  SampleTime=-1
  Integrator t3 : DiscreteIntegrator  ExternalReset=either  InitialCondition=15  InitialConditionSetting=State (most efficient)  SampleTime=-1
  MATLAB Function : MATLAB Function  Priority=1  TreatAsAtomicUnit=on
  Multiport Switch : MultiPortSwitch
  Scope : Scope  NumInputPorts=8
      settings: TickLabels=on  ShowLegends=on  YMin=0~0~0~10~1~1~0~-1  YMax=40~20~20~30~3~3~1~1
  THR1 : Constant  Value=5
  THR2 : Constant  Value=15
  THR3 : Constant  Value=25
  q : Memory  X0=1  LinearizeMemory=on
  reset : Memory  X0=1  LinearizeMemory=on
  state : Outport
  wires:
  MATLAB Function/1(qNext) -> q/1, Scope/6  "q_before"
  Constant/1 -> Integrator t2/1, Integrator t3/1, Integrator t1/1  "y_dot"
  Integrator t2/1 -> Multiport Switch/3, Scope/3
  Integrator t1/1 -> Scope/2, Multiport Switch/2
  THR1/1 -> MATLAB Function/3(THR1)
  THR2/1 -> MATLAB Function/4(THR2)
  q/1 -> Multiport Switch/1, MATLAB Function/2(q), Scope/5  "q_after"
  THR3/1 -> MATLAB Function/5(THR3)
  Integrator t3/1 -> Multiport Switch/4, Scope/4
  MATLAB Function/2(Reset) -> reset/1  "reset_before"
  Multiport Switch/1 -> Scope/1, MATLAB Function/1(y)  "y"
  reset/1 -> Integrator t1/2, Integrator t2/2, Integrator t3/2, Scope/7  "reset_after"
  MATLAB Function/3(gateReq) -> Scope/8, state/1  "gateReq"

== system trainGate/Train25 ==
  Constant : Constant
  Integrator t1 : DiscreteIntegrator  ExternalReset=either  InitialConditionSetting=State (most efficient)  SampleTime=-1
  Integrator t2 : DiscreteIntegrator  ExternalReset=either  InitialCondition=5  InitialConditionSetting=State (most efficient)  SampleTime=-1
  Integrator t3 : DiscreteIntegrator  ExternalReset=either  InitialCondition=15  InitialConditionSetting=State (most efficient)  SampleTime=-1
  MATLAB Function : MATLAB Function  Priority=1  TreatAsAtomicUnit=on
  Multiport Switch : MultiPortSwitch
  Scope : Scope  NumInputPorts=8
      settings: TickLabels=on  ShowLegends=on  YMin=0~0~0~10~1~1~0~-1  YMax=40~20~20~30~3~3~1~1
  THR1 : Constant  Value=5
  THR2 : Constant  Value=15
  THR3 : Constant  Value=25
  q : Memory  X0=1  LinearizeMemory=on
  reset : Memory  X0=1  LinearizeMemory=on
  state : Outport
  wires:
  MATLAB Function/1(qNext) -> q/1, Scope/6  "q_before"
  Constant/1 -> Integrator t2/1, Integrator t3/1, Integrator t1/1  "y_dot"
  Integrator t2/1 -> Multiport Switch/3, Scope/3
  Integrator t1/1 -> Scope/2, Multiport Switch/2
  THR1/1 -> MATLAB Function/3(THR1)
  THR2/1 -> MATLAB Function/4(THR2)
  q/1 -> Multiport Switch/1, MATLAB Function/2(q), Scope/5  "q_after"
  THR3/1 -> MATLAB Function/5(THR3)
  Integrator t3/1 -> Multiport Switch/4, Scope/4
  MATLAB Function/2(Reset) -> reset/1  "reset_before"
  Multiport Switch/1 -> Scope/1, MATLAB Function/1(y)  "y"
  reset/1 -> Integrator t1/2, Integrator t2/2, Integrator t3/2, Scope/7  "reset_after"
  MATLAB Function/3(gateReq) -> Scope/8, state/1  "gateReq"

== system trainGate/Train26 ==
  Constant : Constant
  Integrator t1 : DiscreteIntegrator  ExternalReset=either  InitialConditionSetting=State (most efficient)  SampleTime=-1
  Integrator t2 : DiscreteIntegrator  ExternalReset=either  InitialCondition=5  InitialConditionSetting=State (most efficient)  SampleTime=-1
  Integrator t3 : DiscreteIntegrator  ExternalReset=either  InitialCondition=15  InitialConditionSetting=State (most efficient)  SampleTime=-1
  MATLAB Function : MATLAB Function  Priority=1  TreatAsAtomicUnit=on
  Multiport Switch : MultiPortSwitch
  Scope : Scope  NumInputPorts=8
      settings: TickLabels=on  ShowLegends=on  YMin=0~0~0~10~1~1~0~-1  YMax=40~20~20~30~3~3~1~1
  THR1 : Constant  Value=5
  THR2 : Constant  Value=15
  THR3 : Constant  Value=25
  q : Memory  X0=1  LinearizeMemory=on
  reset : Memory  X0=1  LinearizeMemory=on
  state : Outport
  wires:
  MATLAB Function/1(qNext) -> q/1, Scope/6  "q_before"
  Constant/1 -> Integrator t2/1, Integrator t3/1, Integrator t1/1  "y_dot"
  Integrator t2/1 -> Multiport Switch/3, Scope/3
  Integrator t1/1 -> Scope/2, Multiport Switch/2
  THR1/1 -> MATLAB Function/3(THR1)
  THR2/1 -> MATLAB Function/4(THR2)
  q/1 -> Multiport Switch/1, MATLAB Function/2(q), Scope/5  "q_after"
  THR3/1 -> MATLAB Function/5(THR3)
  Integrator t3/1 -> Multiport Switch/4, Scope/4
  MATLAB Function/2(Reset) -> reset/1  "reset_before"
  Multiport Switch/1 -> Scope/1, MATLAB Function/1(y)  "y"
  reset/1 -> Integrator t1/2, Integrator t2/2, Integrator t3/2, Scope/7  "reset_after"
  MATLAB Function/3(gateReq) -> Scope/8, state/1  "gateReq"

== system trainGate/Train27 ==
  Constant : Constant
  Integrator t1 : DiscreteIntegrator  ExternalReset=either  InitialConditionSetting=State (most efficient)  SampleTime=-1
  Integrator t2 : DiscreteIntegrator  ExternalReset=either  InitialCondition=5  InitialConditionSetting=State (most efficient)  SampleTime=-1
  Integrator t3 : DiscreteIntegrator  ExternalReset=either  InitialCondition=15  InitialConditionSetting=State (most efficient)  SampleTime=-1
  MATLAB Function : MATLAB Function  Priority=1  TreatAsAtomicUnit=on
  Multiport Switch : MultiPortSwitch
  Scope : Scope  NumInputPorts=8
      settings: TickLabels=on  ShowLegends=on  YMin=0~0~0~10~1~1~0~-1  YMax=40~20~20~30~3~3~1~1
  THR1 : Constant  Value=5
  THR2 : Constant  Value=15
  THR3 : Constant  Value=25
  q : Memory  X0=1  LinearizeMemory=on
  reset : Memory  X0=1  LinearizeMemory=on
  state : Outport
  wires:
  MATLAB Function/1(qNext) -> q/1, Scope/6  "q_before"
  Constant/1 -> Integrator t2/1, Integrator t3/1, Integrator t1/1  "y_dot"
  Integrator t2/1 -> Multiport Switch/3, Scope/3
  Integrator t1/1 -> Scope/2, Multiport Switch/2
  THR1/1 -> MATLAB Function/3(THR1)
  THR2/1 -> MATLAB Function/4(THR2)
  q/1 -> Multiport Switch/1, MATLAB Function/2(q), Scope/5  "q_after"
  THR3/1 -> MATLAB Function/5(THR3)
  Integrator t3/1 -> Multiport Switch/4, Scope/4
  MATLAB Function/2(Reset) -> reset/1  "reset_before"
  Multiport Switch/1 -> Scope/1, MATLAB Function/1(y)  "y"
  reset/1 -> Integrator t1/2, Integrator t2/2, Integrator t3/2, Scope/7  "reset_after"
  MATLAB Function/3(gateReq) -> Scope/8, state/1  "gateReq"

== system trainGate/Train28 ==
  Constant : Constant
  Integrator t1 : DiscreteIntegrator  ExternalReset=either  InitialConditionSetting=State (most efficient)  SampleTime=-1
  Integrator t2 : DiscreteIntegrator  ExternalReset=either  InitialCondition=5  InitialConditionSetting=State (most efficient)  SampleTime=-1
  Integrator t3 : DiscreteIntegrator  ExternalReset=either  InitialCondition=15  InitialConditionSetting=State (most efficient)  SampleTime=-1
  MATLAB Function : MATLAB Function  Priority=1  TreatAsAtomicUnit=on
  Multiport Switch : MultiPortSwitch
  Scope : Scope  NumInputPorts=8
      settings: TickLabels=on  ShowLegends=on  YMin=0~0~0~10~1~1~0~-1  YMax=40~20~20~30~3~3~1~1
  THR1 : Constant  Value=5
  THR2 : Constant  Value=15
  THR3 : Constant  Value=25
  q : Memory  X0=1  LinearizeMemory=on
  reset : Memory  X0=1  LinearizeMemory=on
  state : Outport
  wires:
  MATLAB Function/1(qNext) -> q/1, Scope/6  "q_before"
  Constant/1 -> Integrator t2/1, Integrator t3/1, Integrator t1/1  "y_dot"
  Integrator t2/1 -> Multiport Switch/3, Scope/3
  Integrator t1/1 -> Scope/2, Multiport Switch/2
  THR1/1 -> MATLAB Function/3(THR1)
  THR2/1 -> MATLAB Function/4(THR2)
  q/1 -> Multiport Switch/1, MATLAB Function/2(q), Scope/5  "q_after"
  THR3/1 -> MATLAB Function/5(THR3)
  Integrator t3/1 -> Multiport Switch/4, Scope/4
  MATLAB Function/2(Reset) -> reset/1  "reset_before"
  Multiport Switch/1 -> Scope/1, MATLAB Function/1(y)  "y"
  reset/1 -> Integrator t1/2, Integrator t2/2, Integrator t3/2, Scope/7  "reset_after"
  MATLAB Function/3(gateReq) -> Scope/8, state/1  "gateReq"

== system trainGate/Train29 ==
  Constant : Constant
  Integrator t1 : DiscreteIntegrator  ExternalReset=either  InitialConditionSetting=State (most efficient)  SampleTime=-1
  Integrator t2 : DiscreteIntegrator  ExternalReset=either  InitialCondition=5  InitialConditionSetting=State (most efficient)  SampleTime=-1
  Integrator t3 : DiscreteIntegrator  ExternalReset=either  InitialCondition=15  InitialConditionSetting=State (most efficient)  SampleTime=-1
  MATLAB Function : MATLAB Function  Priority=1  TreatAsAtomicUnit=on
  Multiport Switch : MultiPortSwitch
  Scope : Scope  NumInputPorts=8
      settings: TickLabels=on  ShowLegends=on  YMin=0~0~0~10~1~1~0~-1  YMax=40~20~20~30~3~3~1~1
  THR1 : Constant  Value=5
  THR2 : Constant  Value=15
  THR3 : Constant  Value=25
  q : Memory  X0=1  LinearizeMemory=on
  reset : Memory  X0=1  LinearizeMemory=on
  state : Outport
  wires:
  MATLAB Function/1(qNext) -> q/1, Scope/6  "q_before"
  Constant/1 -> Integrator t2/1, Integrator t3/1, Integrator t1/1  "y_dot"
  Integrator t2/1 -> Multiport Switch/3, Scope/3
  Integrator t1/1 -> Scope/2, Multiport Switch/2
  THR1/1 -> MATLAB Function/3(THR1)
  THR2/1 -> MATLAB Function/4(THR2)
  q/1 -> Multiport Switch/1, MATLAB Function/2(q), Scope/5  "q_after"
  THR3/1 -> MATLAB Function/5(THR3)
  Integrator t3/1 -> Multiport Switch/4, Scope/4
  MATLAB Function/2(Reset) -> reset/1  "reset_before"
  Multiport Switch/1 -> Scope/1, MATLAB Function/1(y)  "y"
  reset/1 -> Integrator t1/2, Integrator t2/2, Integrator t3/2, Scope/7  "reset_after"
  MATLAB Function/3(gateReq) -> Scope/8, state/1  "gateReq"

== system trainGate/Train3 ==
  Constant : Constant
  Integrator t1 : DiscreteIntegrator  ExternalReset=either  InitialConditionSetting=State (most efficient)  SampleTime=-1
  Integrator t2 : DiscreteIntegrator  ExternalReset=either  InitialCondition=5  InitialConditionSetting=State (most efficient)  SampleTime=-1
  Integrator t3 : DiscreteIntegrator  ExternalReset=either  InitialCondition=15  InitialConditionSetting=State (most efficient)  SampleTime=-1
  MATLAB Function : MATLAB Function  Priority=1  TreatAsAtomicUnit=on
  Multiport Switch : MultiPortSwitch
  Scope : Scope  NumInputPorts=8
      settings: TickLabels=on  ShowLegends=on  YMin=0~0~0~10~1~1~0~-1  YMax=40~20~20~30~3~3~1~1
  THR1 : Constant  Value=5
  THR2 : Constant  Value=15
  THR3 : Constant  Value=25
  q : Memory  X0=1  LinearizeMemory=on
  reset : Memory  X0=1  LinearizeMemory=on
  state : Outport
  wires:
  MATLAB Function/1(qNext) -> q/1, Scope/6  "q_before"
  Constant/1 -> Integrator t2/1, Integrator t3/1, Integrator t1/1  "y_dot"
  Integrator t2/1 -> Multiport Switch/3, Scope/3
  Integrator t1/1 -> Scope/2, Multiport Switch/2
  THR1/1 -> MATLAB Function/3(THR1)
  THR2/1 -> MATLAB Function/4(THR2)
  q/1 -> Multiport Switch/1, MATLAB Function/2(q), Scope/5  "q_after"
  THR3/1 -> MATLAB Function/5(THR3)
  Integrator t3/1 -> Multiport Switch/4, Scope/4
  MATLAB Function/2(Reset) -> reset/1  "reset_before"
  Multiport Switch/1 -> Scope/1, MATLAB Function/1(y)  "y"
  reset/1 -> Integrator t1/2, Integrator t2/2, Integrator t3/2, Scope/7  "reset_after"
  MATLAB Function/3(gateReq) -> Scope/8, state/1  "gateReq"

== system trainGate/Train4 ==
  Constant : Constant
  Integrator t1 : DiscreteIntegrator  ExternalReset=either  InitialConditionSetting=State (most efficient)  SampleTime=-1
  Integrator t2 : DiscreteIntegrator  ExternalReset=either  InitialCondition=5  InitialConditionSetting=State (most efficient)  SampleTime=-1
  Integrator t3 : DiscreteIntegrator  ExternalReset=either  InitialCondition=15  InitialConditionSetting=State (most efficient)  SampleTime=-1
  MATLAB Function : MATLAB Function  Priority=1  TreatAsAtomicUnit=on
  Multiport Switch : MultiPortSwitch
  Scope : Scope  NumInputPorts=8
      settings: TickLabels=on  ShowLegends=on  YMin=0~0~0~10~1~1~0~-1  YMax=40~20~20~30~3~3~1~1
  THR1 : Constant  Value=5
  THR2 : Constant  Value=15
  THR3 : Constant  Value=25
  q : Memory  X0=1  LinearizeMemory=on
  reset : Memory  X0=1  LinearizeMemory=on
  state : Outport
  wires:
  MATLAB Function/1(qNext) -> q/1, Scope/6  "q_before"
  Constant/1 -> Integrator t2/1, Integrator t3/1, Integrator t1/1  "y_dot"
  Integrator t2/1 -> Multiport Switch/3, Scope/3
  Integrator t1/1 -> Scope/2, Multiport Switch/2
  THR1/1 -> MATLAB Function/3(THR1)
  THR2/1 -> MATLAB Function/4(THR2)
  q/1 -> Multiport Switch/1, MATLAB Function/2(q), Scope/5  "q_after"
  THR3/1 -> MATLAB Function/5(THR3)
  Integrator t3/1 -> Multiport Switch/4, Scope/4
  MATLAB Function/2(Reset) -> reset/1  "reset_before"
  Multiport Switch/1 -> Scope/1, MATLAB Function/1(y)  "y"
  reset/1 -> Integrator t1/2, Integrator t2/2, Integrator t3/2, Scope/7  "reset_after"
  MATLAB Function/3(gateReq) -> Scope/8, state/1  "gateReq"

== system trainGate/Train5 ==
  Constant : Constant
  Integrator t1 : DiscreteIntegrator  ExternalReset=either  InitialConditionSetting=State (most efficient)  SampleTime=-1
  Integrator t2 : DiscreteIntegrator  ExternalReset=either  InitialCondition=5  InitialConditionSetting=State (most efficient)  SampleTime=-1
  Integrator t3 : DiscreteIntegrator  ExternalReset=either  InitialCondition=15  InitialConditionSetting=State (most efficient)  SampleTime=-1
  MATLAB Function : MATLAB Function  Priority=1  TreatAsAtomicUnit=on
  Multiport Switch : MultiPortSwitch
  Scope : Scope  NumInputPorts=8
      settings: TickLabels=on  ShowLegends=on  YMin=0~0~0~10~1~1~0~-1  YMax=40~20~20~30~3~3~1~1
  THR1 : Constant  Value=5
  THR2 : Constant  Value=15
  THR3 : Constant  Value=25
  q : Memory  X0=1  LinearizeMemory=on
  reset : Memory  X0=1  LinearizeMemory=on
  state : Outport
  wires:
  MATLAB Function/1(qNext) -> q/1, Scope/6  "q_before"
  Constant/1 -> Integrator t2/1, Integrator t3/1, Integrator t1/1  "y_dot"
  Integrator t2/1 -> Multiport Switch/3, Scope/3
  Integrator t1/1 -> Scope/2, Multiport Switch/2
  THR1/1 -> MATLAB Function/3(THR1)
  THR2/1 -> MATLAB Function/4(THR2)
  q/1 -> Multiport Switch/1, MATLAB Function/2(q), Scope/5  "q_after"
  THR3/1 -> MATLAB Function/5(THR3)
  Integrator t3/1 -> Multiport Switch/4, Scope/4
  MATLAB Function/2(Reset) -> reset/1  "reset_before"
  Multiport Switch/1 -> Scope/1, MATLAB Function/1(y)  "y"
  reset/1 -> Integrator t1/2, Integrator t2/2, Integrator t3/2, Scope/7  "reset_after"
  MATLAB Function/3(gateReq) -> Scope/8, state/1  "gateReq"

== system trainGate/Train6 ==
  Constant : Constant
  Integrator t1 : DiscreteIntegrator  ExternalReset=either  InitialConditionSetting=State (most efficient)  SampleTime=-1
  Integrator t2 : DiscreteIntegrator  ExternalReset=either  InitialCondition=5  InitialConditionSetting=State (most efficient)  SampleTime=-1
  Integrator t3 : DiscreteIntegrator  ExternalReset=either  InitialCondition=15  InitialConditionSetting=State (most efficient)  SampleTime=-1
  MATLAB Function : MATLAB Function  Priority=1  TreatAsAtomicUnit=on
  Multiport Switch : MultiPortSwitch
  Scope : Scope  NumInputPorts=8
      settings: TickLabels=on  ShowLegends=on  YMin=0~0~0~10~1~1~0~-1  YMax=40~20~20~30~3~3~1~1
  THR1 : Constant  Value=5
  THR2 : Constant  Value=15
  THR3 : Constant  Value=25
  q : Memory  X0=1  LinearizeMemory=on
  reset : Memory  X0=1  LinearizeMemory=on
  state : Outport
  wires:
  MATLAB Function/1(qNext) -> q/1, Scope/6  "q_before"
  Constant/1 -> Integrator t2/1, Integrator t3/1, Integrator t1/1  "y_dot"
  Integrator t2/1 -> Multiport Switch/3, Scope/3
  Integrator t1/1 -> Scope/2, Multiport Switch/2
  THR1/1 -> MATLAB Function/3(THR1)
  THR2/1 -> MATLAB Function/4(THR2)
  q/1 -> Multiport Switch/1, MATLAB Function/2(q), Scope/5  "q_after"
  THR3/1 -> MATLAB Function/5(THR3)
  Integrator t3/1 -> Multiport Switch/4, Scope/4
  MATLAB Function/2(Reset) -> reset/1  "reset_before"
  Multiport Switch/1 -> Scope/1, MATLAB Function/1(y)  "y"
  reset/1 -> Integrator t1/2, Integrator t2/2, Integrator t3/2, Scope/7  "reset_after"
  MATLAB Function/3(gateReq) -> Scope/8, state/1  "gateReq"

== system trainGate/Train7 ==
  Constant : Constant
  Integrator t1 : DiscreteIntegrator  ExternalReset=either  InitialConditionSetting=State (most efficient)  SampleTime=-1
  Integrator t2 : DiscreteIntegrator  ExternalReset=either  InitialCondition=5  InitialConditionSetting=State (most efficient)  SampleTime=-1
  Integrator t3 : DiscreteIntegrator  ExternalReset=either  InitialCondition=15  InitialConditionSetting=State (most efficient)  SampleTime=-1
  MATLAB Function : MATLAB Function  Priority=1  TreatAsAtomicUnit=on
  Multiport Switch : MultiPortSwitch
  Scope : Scope  NumInputPorts=8
      settings: TickLabels=on  ShowLegends=on  YMin=0~0~0~10~1~1~0~-1  YMax=40~20~20~30~3~3~1~1
  THR1 : Constant  Value=5
  THR2 : Constant  Value=15
  THR3 : Constant  Value=25
  q : Memory  X0=1  LinearizeMemory=on
  reset : Memory  X0=1  LinearizeMemory=on
  state : Outport
  wires:
  MATLAB Function/1(qNext) -> q/1, Scope/6  "q_before"
  Constant/1 -> Integrator t2/1, Integrator t3/1, Integrator t1/1  "y_dot"
  Integrator t2/1 -> Multiport Switch/3, Scope/3
  Integrator t1/1 -> Scope/2, Multiport Switch/2
  THR1/1 -> MATLAB Function/3(THR1)
  THR2/1 -> MATLAB Function/4(THR2)
  q/1 -> Multiport Switch/1, MATLAB Function/2(q), Scope/5  "q_after"
  THR3/1 -> MATLAB Function/5(THR3)
  Integrator t3/1 -> Multiport Switch/4, Scope/4
  MATLAB Function/2(Reset) -> reset/1  "reset_before"
  Multiport Switch/1 -> Scope/1, MATLAB Function/1(y)  "y"
  reset/1 -> Integrator t1/2, Integrator t2/2, Integrator t3/2, Scope/7  "reset_after"
  MATLAB Function/3(gateReq) -> Scope/8, state/1  "gateReq"

== system trainGate/Train8 ==
  Constant : Constant
  Integrator t1 : DiscreteIntegrator  ExternalReset=either  InitialConditionSetting=State (most efficient)  SampleTime=-1
  Integrator t2 : DiscreteIntegrator  ExternalReset=either  InitialCondition=5  InitialConditionSetting=State (most efficient)  SampleTime=-1
  Integrator t3 : DiscreteIntegrator  ExternalReset=either  InitialCondition=15  InitialConditionSetting=State (most efficient)  SampleTime=-1
  MATLAB Function : MATLAB Function  Priority=1  TreatAsAtomicUnit=on
  Multiport Switch : MultiPortSwitch
  Scope : Scope  NumInputPorts=8
      settings: TickLabels=on  ShowLegends=on  YMin=0~0~0~10~1~1~0~-1  YMax=40~20~20~30~3~3~1~1
  THR1 : Constant  Value=5
  THR2 : Constant  Value=15
  THR3 : Constant  Value=25
  q : Memory  X0=1  LinearizeMemory=on
  reset : Memory  X0=1  LinearizeMemory=on
  state : Outport
  wires:
  MATLAB Function/1(qNext) -> q/1, Scope/6  "q_before"
  Constant/1 -> Integrator t2/1, Integrator t3/1, Integrator t1/1  "y_dot"
  Integrator t2/1 -> Multiport Switch/3, Scope/3
  Integrator t1/1 -> Scope/2, Multiport Switch/2
  THR1/1 -> MATLAB Function/3(THR1)
  THR2/1 -> MATLAB Function/4(THR2)
  q/1 -> Multiport Switch/1, MATLAB Function/2(q), Scope/5  "q_after"
  THR3/1 -> MATLAB Function/5(THR3)
  Integrator t3/1 -> Multiport Switch/4, Scope/4
  MATLAB Function/2(Reset) -> reset/1  "reset_before"
  Multiport Switch/1 -> Scope/1, MATLAB Function/1(y)  "y"
  reset/1 -> Integrator t1/2, Integrator t2/2, Integrator t3/2, Scope/7  "reset_after"
  MATLAB Function/3(gateReq) -> Scope/8, state/1  "gateReq"
